simulink model "detumbling1"  (R2022b)
settings: Solver=ode5  StartTime=startTime  StopTime=stopTime  FixedStep=stepsize  RelTol=1e-3
undefined symbols (not defined in the file): a, A_BN0, ARW, c, detumblingkb, detumblingkp, e, EHAccuracy, EHSampleRate, first_detumbling_time_1RW, G, GyroSampleRate, H, h_RW_max, i, inertia1, inertia2, inertia3, Inertia_matrix, Inverse_inertia, Ld, Lw, m, maxdipole, MB, MMnoise, MMSampleRate, mu, n, R_e, rho_d_MB, rho_d_SP, rho_s_MB, rho_s_SP, RRW, SP, theta0, torque_RW_max, w0, wheel_axis
libraries: matrix_library x11, vrlib x10, simulink_extras x4
(part 1 of 3)
settings Model: Creator=Alessandro Cambielli  LastModifiedBy=Alessandro Cambielli

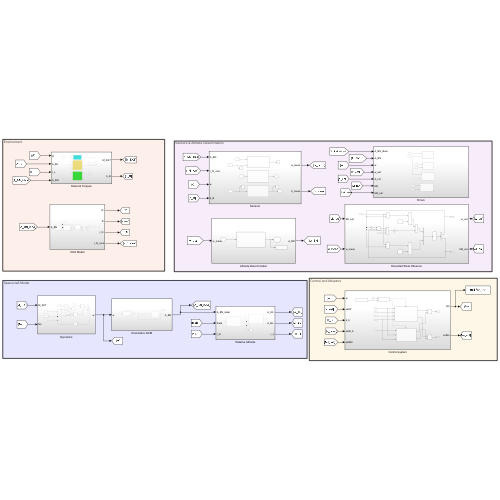
[thumbnail: Simulink's stored preview of the top-level diagram]
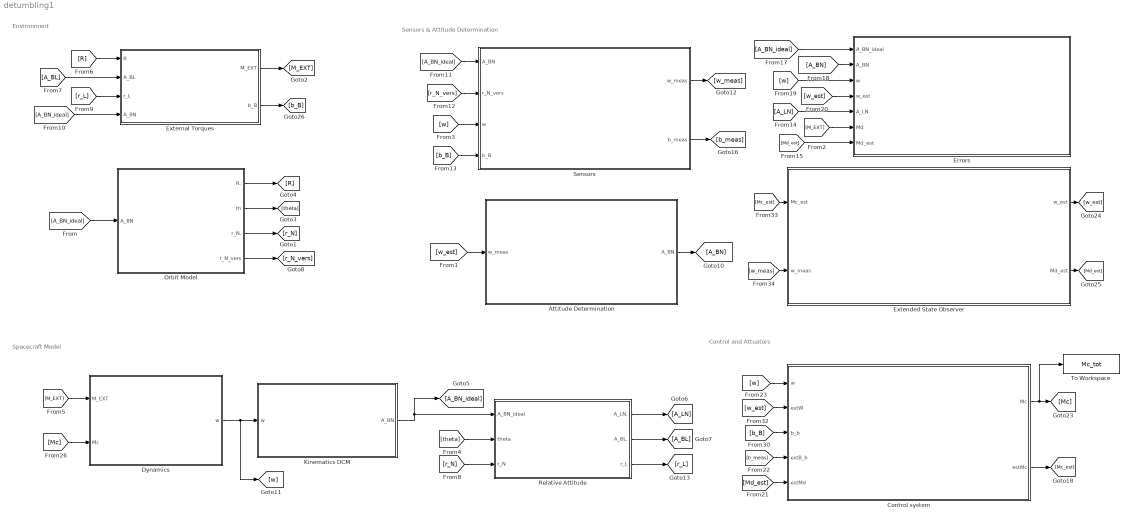
== system detumbling1 ==
  note: Control and Attuators
  note: Sensors & Attitude Determination
  note: Environment
  note: Spacecraft Model
  Attitude Determination : Subsystem
  Control system : Subsystem
  Dynamics : Subsystem
  Errors : Subsystem
  Extended State Observer : Subsystem
  External Torques : Subsystem
  Kinematics DCM : Subsystem
  Orbit Model : Subsystem
  Relative Attitude : Subsystem
  Sensors : Subsystem
  To Workspace : ToWorkspace  VariableName=Mc_tot  SaveFormat=Timeseries  SampleTime=-1
  wires:
  External Torques/2(b_B) -> [b_B]
  [w_est] -> Errors/4(w_est)
  Kinematics DCM/1(A_BN) -> Relative Attitude/1(A_BN_ideal), [A_BN_ideal]
  [w_est] -> Attitude Determination/1(w_meas)
  [M_EXT] -> Errors/6(Md)
  [A_BL] -> External Torques/2(A_BL)
  [Md_est] -> Errors/7(Md_est)
  Orbit Model/3(r_N.) -> [r_N]
  Relative Attitude/2(A_BL.) -> [A_BL]
  Sensors/1(w_meas) -> [w_meas]
  External Torques/1(M_EXT) -> [M_EXT]
  [M_EXT] -> Dynamics/1(M_EXT)
  [A_BN_ideal] -> Orbit Model/1(A_BN)
  Relative Attitude/1(A_LN.) -> [A_LN]
  Sensors/2(b_meas) -> [b_meas]
  [b_B] -> Control system/3(b_b)
  [w_est] -> Control system/2(estW)
  Orbit Model/2(th) -> [theta]
  [A_BN_ideal] -> Errors/1(A_BN_ideal)
  Orbit Model/4(r_N_vers) -> [r_N_vers]
  [r_N_vers] -> Sensors/2(r_N_vers)
  [w_meas] -> Extended State Observer/2(w_meas)
  [r_N] -> Relative Attitude/3(r_N)
  [Md_est] -> Control system/5(estMd)
  Extended State Observer/2(Md_est) -> [Md_est]
  [w] -> Control system/1(w)
  Dynamics/1(w) -> [w], Kinematics DCM/1(w)
  Orbit Model/1(R.) -> [R]
  Control system/2(estMc) -> [Mc_est]
  Control system/1(Mc) -> To Workspace/1, [Mc]
  Relative Attitude/3(r_L) -> [r_L]
  Extended State Observer/1(w_est) -> [w_est]
  [A_BN_ideal] -> Sensors/1(A_BN)
  [A_BN] -> Errors/2(A_BN)
  [A_BN_ideal] -> External Torques/4(A_BN)
  [w] -> Sensors/3(w)
  Attitude Determination/1(A_BN) -> [A_BN]
  [R] -> External Torques/1(R)
  [theta] -> Relative Attitude/2(theta)
  [A_LN] -> Errors/5(A_LN)
  [b_meas] -> Control system/4(estB_b)
  [b_B] -> Sensors/4(b_B)
  [Mc_est] -> Extended State Observer/1(Mc_est)
  [r_L] -> External Torques/3(r_L)
  [w] -> Errors/3(w)
  [Mc] -> Dynamics/2(Mc)

== system detumbling1/Attitude Determination ==
  w_meas : Inport
  Kinematics DCM1 : Subsystem
  To Workspace : ToWorkspace  VariableName=A_BN  SampleTime=-1
  A_BN : Outport
  wires:
  w_meas/1 -> Kinematics DCM1/1(w)
  Kinematics DCM1/1(A_BN) -> To Workspace/1, A_BN/1

== system detumbling1/Control system ==
  w : Inport
  estW : Inport  Port=2
  b_b : Inport  Port=3
  estB_b : Inport  Port=4
  estMd : Inport  Port=5
  Clock : Clock
  Constant : Constant  Value=first_detumbling_time_1RW
  If : If  NumInputs=2  IfExpression=u1 <= u2
  Merge : Merge
  Merge1 : Merge
  Proportional control (RWs) : Subsystem  TreatAsAtomicUnit=on
  Spin rate damping (MT) : Subsystem  TreatAsAtomicUnit=on
  Mc : Outport
  estMc : Outport  Port=2
  wires:
  b_b/1 -> Spin rate damping (MT)/2(b_b)
  Spin rate damping (MT)/1(Mc) -> Merge/1
  Constant/1 -> If/2
  Spin rate damping (MT)/2(estMc) -> Merge1/1
  Proportional control (RWs)/1(Mc) -> Merge/2
  Merge/1 -> Mc/1
  Merge1/1 -> estMc/1
  estB_b/1 -> Spin rate damping (MT)/3(estB_b)
  Clock/1 -> If/1
  estMd/1 -> Proportional control (RWs)/3(estMd), Spin rate damping (MT)/4(estMd)
  If/2 -> Proportional control (RWs)/Action
  estW/1 -> Proportional control (RWs)/2(estW), Spin rate damping (MT)/1(estW)
  If/1 -> Spin rate damping (MT)/Action
  w/1 -> Proportional control (RWs)/1(w)
  Proportional control (RWs)/2(estMc) -> Merge1/2

== system detumbling1/Dynamics ==
  M_EXT : Inport
  Mc : Inport  Port=2
  Constant : Constant  Value=Inverse_inertia
  Constant1 : Constant  Value=Inertia_matrix
  Constant2 : Constant  Value=Inverse_inertia
  Cross Product : matrix_library/Cross Product
  Integrator : Integrator  InitialCondition=w0
  MatrixMultiply : Product  Multiplication=Matrix(*)
  MatrixMultiply1 : Product  Multiplication=Matrix(*)
  MatrixMultiply2 : Product  Multiplication=Matrix(*)
  Scope : Scope
  Sum : Sum
  Sum1 : Sum
  To Workspace : ToWorkspace  VariableName=w  SaveFormat=Timeseries  SampleTime=-1
  w : Outport
  wires:
  MatrixMultiply2/1 -> Sum1/2
  Sum1/1 -> Integrator/1
  Integrator/1 -> w/1, Cross Product/2, Scope/1, To Workspace/1, MatrixMultiply1/2
  Constant/1 -> MatrixMultiply/1
  Constant2/1 -> MatrixMultiply2/1
  MatrixMultiply/1 -> Sum1/1
  Constant1/1 -> MatrixMultiply1/1
  Cross Product/1 -> MatrixMultiply/2
  MatrixMultiply1/1 -> Cross Product/1
  Sum/1 -> MatrixMultiply2/2
  M_EXT/1 -> Sum/1
  Mc/1 -> Sum/2

== system detumbling1/Errors ==
  A_BN_ideal : Inport
  A_BN : Inport  Port=2
  w : Inport  Port=3
  w_est : Inport  Port=4
  A_LN : Inport  Port=5
  Md : Inport  Port=6
  Md_est : Inport  Port=7
  Md error : Subsystem
  Subsystem : Subsystem
  omega error : Subsystem
  pointing error : Subsystem
  wires:
  w/1 -> omega error/1(w)
  w_est/1 -> omega error/2(w_meas)
  A_BN_ideal/1 -> Subsystem/1(A_BN_ideal)
  A_BN/1 -> Subsystem/2(A_BN), pointing error/1(A_BN)
  A_LN/1 -> pointing error/2(A_LN)
  Md/1 -> Md error/1(Md)
  Md_est/1 -> Md error/2(Md_est)

== system detumbling1/Extended State Observer ==
  Mc_est : Inport
  w_meas : Inport  Port=2
  Constant4 : Constant  Value=Lw
  Constant5 : Constant  Value=Ld
  Cross Product : vrlib/Utilities/Cross Product
  Demux1 : Demux  Outputs=2
  Gain : Gain  Gain=Inertia_matrix  Multiplication=Matrix(K*u)
  Gain1 : Gain  Gain=Inverse_inertia  Multiplication=Matrix(K*u)
  Integrator : Integrator  InitialCondition=[w0; [0; 0; 0]]
  Mux : Mux  Inputs=2
  Product4 : Product
  Product5 : Product
  Sum4 : Sum  Inputs=+-
  Sum5 : Sum  Inputs=+-
  Sum6 : Sum
  Sum7 : Sum  Inputs=+++
  w_est : Outport
  Md_est : Outport  Port=2
  wires:
  Gain/1 -> Cross Product/1
  Sum5/1 -> Product5/1
  Constant5/1 -> Product5/2
  Cross Product/1 -> Sum7/1
  Product5/1 -> Mux/2
  Demux1/1 -> Sum5/2, Cross Product/2, Gain/1, Sum4/2, w_est/1
  Sum7/1 -> Gain1/1
  Gain1/1 -> Sum6/2
  Product4/1 -> Sum6/1
  Sum6/1 -> Mux/1
  Demux1/2 -> Md_est/1, Sum7/2
  Mux/1 -> Integrator/1
  Mc_est/1 -> Sum7/3
  w_meas/1 -> Sum5/1, Sum4/1
  Integrator/1 -> Demux1/1
  Constant4/1 -> Product4/2
  Sum4/1 -> Product4/1

== system detumbling1/External Torques ==
  R : Inport
  A_BL : Inport  Port=2
  r_L : Inport  Port=3
  A_BN : Inport  Port=4
  Constant : Constant  Value=MB
  Constant1 : Constant  Value=SP
  M_GG : Subsystem
  Magnetic field : Subsystem
  Solar radiation : Subsystem
  Sum of Elements : Sum  Inputs=+++
  To Workspace : ToWorkspace  VariableName=M_GG  SaveFormat=Timeseries  SampleTime=-1
  To Workspace1 : ToWorkspace  VariableName=M_SRP  SaveFormat=Timeseries  SampleTime=-1
  To Workspace2 : ToWorkspace  VariableName=M_MAG  SaveFormat=Timeseries  SampleTime=-1
  M_EXT : Outport
  b_B : Outport  Port=2
  wires:
  [R] -> M_GG/2(R)
  Constant/1 -> Solar radiation/2(MB)
  Constant1/1 -> Solar radiation/3(SP)
  [A_BN] -> Solar radiation/1(A_BN)
  [A_BN] -> Magnetic field/2(A_BN)
  Magnetic field/1(M_MAG) -> Sum of Elements/3, To Workspace2/1
  Sum of Elements/1 -> M_EXT/1
  [A_BL] -> M_GG/1(A_BL)
  [r_L] -> Magnetic field/1(r_L)
  R/1 -> [R]
  A_BL/1 -> [A_BL]
  M_GG/1(M_GG1) -> Sum of Elements/1, To Workspace/1
  r_L/1 -> [r_L]
  A_BN/1 -> [A_BN]
  Solar radiation/1(T_SRP) -> To Workspace1/1, Sum of Elements/2
  Magnetic field/2(b_B) -> b_B/1

== system detumbling1/Kinematics DCM ==
  w : Inport
  Gain : Gain  Gain=-1
  Integrator : Integrator  InitialCondition=A_BN0
  Product : Product  Multiplication=Matrix(*)
  To Workspace : ToWorkspace  VariableName=A_BN_ideal  SampleTime=-1
  orthonormalization : Subsystem
  w_cross : Subsystem
  A_BN : Outport
  wires:
  w_cross/1(w_cross) -> Gain/1
  Product/1 -> Integrator/1
  Gain/1 -> Product/1
  Integrator/1 -> orthonormalization/1(A0(t))
  orthonormalization/1(A(t)) -> A_BN/1, To Workspace/1, Product/2
  w/1 -> w_cross/1(w)

== system detumbling1/Orbit Model ==
  A_BN : Inport
  Normalize Vector : vrlib/Utilities/Normalize Vector  maxzero=0
  Product : Product  Multiplication=Matrix(*)
  R : Subsystem
  To Workspace1 : ToWorkspace  VariableName=r_B_vers  SampleTime=-1
  r_N : Subsystem
  theta : Subsystem
  R. : Outport
  th : Outport  Port=2
  r_N. : Outport  Port=3
  r_N_vers : Outport  Port=4
  wires:
  Normalize Vector/1 -> r_N_vers/1, Product/2
  r_N/1(r_N) -> r_N./1, Normalize Vector/1
  R/1(R) -> R./1, r_N/2(R)
  Product/1 -> To Workspace1/1
  theta/1(theta) -> th/1, r_N/1(theta), R/1(theta)
  A_BN/1 -> Product/1

== system detumbling1/Relative Attitude ==
  A_BN_ideal : Inport
  theta : Inport  Port=2
  r_N : Inport  Port=3
  A_BL : Subsystem
  A_LN : Subsystem
  MatrixMultiply : Product  Multiplication=Matrix(*)
  A_LN. : Outport
  A_BL. : Outport  Port=2
  r_L : Outport  Port=3
  wires:
  A_LN/1(A_LN) -> MatrixMultiply/1, A_LN./1, A_BL/2(A_LN)
  theta/1 -> A_LN/1(theta)
  A_BN_ideal/1 -> A_BL/1(A_BN)
  A_BL/1(A_BL) -> A_BL./1
  r_N/1 -> MatrixMultiply/2
  MatrixMultiply/1 -> r_L/1

== system detumbling1/Sensors ==
  A_BN : Inport
  r_N_vers : Inport  Port=2
  w : Inport  Port=3
  b_B : Inport  Port=4
  Earth Horizon Sensor : Subsystem
  Gyroscope : Subsystem
  Magnetometer : Subsystem
  Scope{,1..3} (4 alike) : Scope
  w_meas : Outport
  b_meas : Outport  Port=2
  wires:
  A_BN/1 -> Earth Horizon Sensor/1(A_BN)
  r_N_vers/1 -> Scope/1, Earth Horizon Sensor/2(r_N_vers)
  w/1 -> Gyroscope/1(w)
  b_B/1 -> Scope2/1, Magnetometer/1(b_B)
  Earth Horizon Sensor/1(EH_meas) -> Scope1/1
  Gyroscope/1(w_meas) -> w_meas/1
  Magnetometer/1(MM_meas) -> Scope3/1, b_meas/1

== system detumbling1/Attitude Determination/Kinematics DCM1 ==
  w : Inport
  Gain : Gain  Gain=-1
  Integrator : Integrator  InitialCondition=A_BN0
  Product : Product  Multiplication=Matrix(*)
  orthonormalization : Subsystem
  w_cross : Subsystem
  A_BN : Outport
  wires:
  w_cross/1(w_cross) -> Gain/1
  Product/1 -> Integrator/1
  Gain/1 -> Product/1
  Integrator/1 -> orthonormalization/1(A0(t))
  orthonormalization/1(A(t)) -> A_BN/1, Product/2
  w/1 -> w_cross/1(w)

== system detumbling1/Control system/Proportional control (RWs) ==
  w : Inport
  estW : Inport  Port=2
  estMd : Inport  Port=3
  Action Port : ActionPort  ActionPortLabel=else
  Ideal control law : Subsystem  TreatAsAtomicUnit=on
  Reaction wheels : Subsystem
  Scope : Scope
  To Workspace : ToWorkspace  VariableName=Mc_RW  SaveFormat=Timeseries  SampleTime=-1
  Mc : Outport
  estMc : Outport  Port=2
  wires:
  Reaction wheels/2(estMc_RW) -> estMc/1
  Ideal control law/1(Mc_id) -> Reaction wheels/1(targetMc)
  w/1 -> Reaction wheels/2(w)
  estW/1 -> Reaction wheels/3(estW), Ideal control law/1(estW)
  estMd/1 -> Ideal control law/2(estMd)
  Reaction wheels/1(Mc_RW) -> To Workspace/1, Scope/1, Mc/1

== system detumbling1/Control system/Spin rate damping (MT) ==
  estW : Inport
  b_b : Inport  Port=2
  estB_b : Inport  Port=3
  estMd : Inport  Port=4
  Action Port : ActionPort  ActionPortLabel=if(u1 <= u2)
  Ideal control law : Subsystem
  Magnetorquer : Subsystem
  Scope : Scope
  To Workspace : ToWorkspace  VariableName=Mc_MT  SaveFormat=Timeseries  SampleTime=-1
  Mc : Outport
  estMc : Outport  Port=2
  wires:
  b_b/1 -> Magnetorquer/2(b_b)
  estB_b/1 -> Magnetorquer/3(estB_b), Ideal control law/2(estB_b)
  Ideal control law/1(targetMc) -> Magnetorquer/1(targetMc)
  Magnetorquer/1(Mc_MT) -> Scope/1, To Workspace/1, Mc/1
  estMd/1 -> Ideal control law/3(estMd)
  estW/1 -> Ideal control law/1(estW)
  Magnetorquer/2(estMc_MT) -> estMc/1

== system detumbling1/Errors/Md error ==
  Md : Inport
  Md_est : Inport  Port=2
  Scope2 : Scope
  Sum : Sum  Inputs=+-
  To Workspace1 : ToWorkspace  VariableName=delta_Md  SaveFormat=Timeseries  SampleTime=-1
  wires:
  Sum/1 -> Scope2/1, To Workspace1/1
  Md/1 -> Sum/1
  Md_est/1 -> Sum/2

== system detumbling1/Errors/Subsystem ==
  A_BN_ideal : Inport
  A_BN : Inport  Port=2
  Acos : Trigonometry  Commented=on  Operator=acos
  Acos1 : Trigonometry  Commented=on  Operator=acos
  Constant : Constant  Value=eye(3)
  Gain : Gain  Commented=on  Gain=2
  Gain1 : Gain  Commented=on  Gain=2
  MATLAB Function : MATLAB Function  Commented=on  TreatAsAtomicUnit=on
  MatrixMultiply : Product  Multiplication=Matrix(*)
  Radians to Degrees : simulink_extras/Transformations/Radians to Degrees  Commented=on
  Radians to Degrees1 : simulink_extras/Transformations/Radians to Degrees  Commented=on
  Sum : Sum  Inputs=+-
  Sum1 : Sum  Commented=on  Inputs=+-
  To Workspace : ToWorkspace  VariableName=A_error  SaveFormat=Timeseries  SampleTime=-1
  Transpose : Math  Operator=transpose
  wires:
  MATLAB Function/1(q4) -> Acos/1
  MATLAB Function/2(q4_sens) -> Acos1/1
  Acos/1 -> Gain/1
  Acos1/1 -> Gain1/1
  Gain/1 -> Radians to Degrees/1
  Gain1/1 -> Radians to Degrees1/1
  Radians to Degrees/1 -> Sum1/1
  Radians to Degrees1/1 -> Sum1/2
  A_BN_ideal/1 -> MatrixMultiply/1
  A_BN/1 -> Transpose/1
  Transpose/1 -> MatrixMultiply/2
  MatrixMultiply/1 -> Sum/1
  Constant/1 -> Sum/2
  Sum/1 -> To Workspace/1

== system detumbling1/Errors/omega error ==
  w : Inport
  w_meas : Inport  Port=2
  Scope : Scope
  Sum1 : Sum  Inputs=+-
  To Workspace1 : ToWorkspace  VariableName=delta_omega  SaveFormat=Timeseries  SampleTime=-1
  wires:
  Sum1/1 -> Scope/1, To Workspace1/1
  w/1 -> Sum1/1
  w_meas/1 -> Sum1/2

== system detumbling1/Errors/pointing error ==
  A_BN : Inport
  A_LN : Inport  Port=2
  Constant : Constant  Value=[1; 0; 0]
  Constant1 : Constant  Value=[1; 0; 0]
  Dot Product : DotProduct  OutDataTypeStr=Inherit: Inherit via internal rule
  MatrixMultiply : Product  Inputs=3  Multiplication=Matrix(*)
  Radians to Degrees : simulink_extras/Transformations/Radians to Degrees
  Scope : Scope
  To Workspace : ToWorkspace  VariableName=point_error  SaveFormat=Timeseries  SampleTime=-1
  Transpose1 : matrix_library/Transpose
  Trigonometric Function : Trigonometry  Operator=acos
  wires:
  A_LN/1 -> Transpose1/1
  Trigonometric Function/1 -> Radians to Degrees/1
  A_BN/1 -> MatrixMultiply/1
  Transpose1/1 -> MatrixMultiply/2
  Constant/1 -> MatrixMultiply/3
  MatrixMultiply/1 -> Dot Product/1
  Constant1/1 -> Dot Product/2
  Dot Product/1 -> Trigonometric Function/1
  Radians to Degrees/1 -> Scope/1, To Workspace/1

== system detumbling1/External Torques/M_GG ==
  A_BL : Inport
  R : Inport  Port=2
  GG Torque1 : Subsystem
  "c1, c2, c3" : Subsystem
  M_GG1 : Outport
  wires:
  "c1, c2, c3"/1(c1) -> GG Torque1/1(c1)
  "c1, c2, c3"/2(c2) -> GG Torque1/2(c2)
  "c1, c2, c3"/3(c3) -> GG Torque1/3(c3)
  A_BL/1 -> "c1, c2, c3"/1(A_BL)
  GG Torque1/1(M_GG) -> M_GG1/1
  R/1 -> GG Torque1/4(R)

== system detumbling1/External Torques/Magnetic field ==
  r_L : Inport
  A_BN : Inport  Port=2
  Clock : Clock
  Constant : Constant  Value=m
  Constant1 : Constant  Value=R_e*1000
  Constant3 : Constant  Value=G
  Constant4 : Constant  Value=H
  Cross Product1 : matrix_library/Cross Product
  MATLAB Function : MATLAB Function  TreatAsAtomicUnit=on
  MatrixMultiply : Product  Multiplication=Matrix(*)
  Reshape1 : Reshape  OutputDimensionality=Column vector (2-D)
  M_MAG : Outport
  b_B : Outport  Port=2
  wires:
  Constant1/1 -> MATLAB Function/2(r)
  Clock/1 -> MATLAB Function/3(t)
  Constant3/1 -> MATLAB Function/4(G)
  MATLAB Function/1(b_N) -> Reshape1/1
  r_L/1 -> MATLAB Function/1(r_LVLH)
  Reshape1/1 -> MatrixMultiply/2
  Constant4/1 -> MATLAB Function/5(H)
  A_BN/1 -> MatrixMultiply/1
  Constant/1 -> Cross Product1/1
  MatrixMultiply/1 -> b_B/1, Cross Product1/2
  Cross Product1/1 -> M_MAG/1

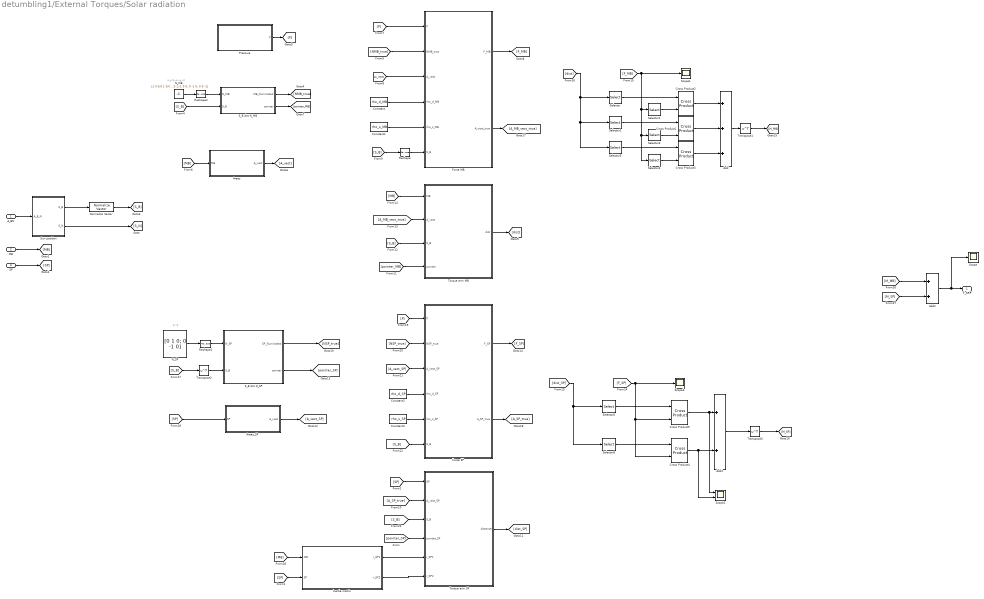
== system detumbling1/External Torques/Solar radiation ==
  note: x,y,z,-x,-y,-z
  note: y,-y
  A_BN : Inport
  MB : Inport  Port=2
  SP : Inport  Port=3
  Add : Sum  Inputs=3
  Add1 : Sum
  Add2 : Sum
  Areas : Subsystem
  Areas_SP : Subsystem
  Constant : Constant  Value=rho_d_MB
  Constant1 : Constant  Value=rho_s_MB
  Constant2 : Constant  Value=rho_d_SP
  Constant3 : Constant  Value=rho_s_SP
  Cross Product{1..5} (5 alike) : matrix_library/Cross Product
  Force MB : Subsystem
  Force SP : Subsystem
  Inertia matrix : Subsystem
  N_MB : Constant  Value=[1 0 0;0 1 0;0 0 1;-1 0 0; 0 -1 0; 0 0 -1]  VectorParams1D=off
  N_SP : Constant  Value=[0 1 0; 0 -1 0]  VectorParams1D=off
  Normalize Vector : vrlib/Utilities/Normalize Vector  maxzero=0
  Pressure : Subsystem
  Reshape : Reshape  OutputDimensionality=Column vector (2-D)
  Reshape1 : Reshape  OutputDimensionality=Customize  OutputDimensions=[2,3]
  Reshape2 : Reshape  OutputDimensionality=Customize  OutputDimensions=[6,3]
  S_B dot N_MB : Subsystem
  S_B dot N_SP : Subsystem
  Scope : Scope
  Scope1 : Scope
  Scope2 : Scope  NumInputPorts=2
  Scope3 : Scope
  Selector : Selector  NumberOfDimensions=2  InputPortWidth=3  IndexOptions=Index vector (dialog),Index vector (dialog)  Indices=1,[1 2 3]  OutputSizes=1,1
  Selector1 : Selector  NumberOfDimensions=2  InputPortWidth=3  IndexOptions=Index vector (dialog),Index vector (dialog)  Indices=1,[1 2 3]  OutputSizes=1,1
  Selector2 : Selector  NumberOfDimensions=2  InputPortWidth=3  IndexOptions=Index vector (dialog),Index vector (dialog)  Indices=2,[1 2 3]  OutputSizes=1,1
  Selector3 : Selector  NumberOfDimensions=2  InputPortWidth=3  IndexOptions=Index vector (dialog),Index vector (dialog)  Indices=2,[1 2 3]  OutputSizes=1,1
  Selector4 : Selector  NumberOfDimensions=2  InputPortWidth=3  IndexOptions=Index vector (dialog),Index vector (dialog)  Indices=3,[1 2 3]  OutputSizes=1,1
  Selector5 : Selector  NumberOfDimensions=2  InputPortWidth=3  IndexOptions=Index vector (dialog),Index vector (dialog)  Indices=3,[1 2 3]  OutputSizes=1,1
  Selector6 : Selector  NumberOfDimensions=2  InputPortWidth=3  IndexOptions=Index vector (dialog),Index vector (dialog)  Indices=1,[1 2 3]  OutputSizes=1,1
  Selector8 : Selector  NumberOfDimensions=2  InputPortWidth=3  IndexOptions=Index vector (dialog),Index vector (dialog)  Indices=2,[1 2 3]  OutputSizes=1,1
  Sun position : Subsystem
  Torque arm MB : Subsystem
  Torque arm SP : Subsystem
  Transpose1 : Math  Operator=transpose
  Transpose2 : Math  Operator=transpose
  Transpose3 : Math  Operator=transpose
  T_SRP : Outport
  wires:
  Sun position/1(S_B) -> Normalize Vector/1
  MB/1 -> [MB]
  N_MB/1 -> Reshape2/1
  [NMB_true] -> Force MB/2(NMB_true)
  S_B dot N_MB/1(MB_illuminated) -> [NMB_true]
  [MB] -> Areas/1(MB)
  [S_B] -> S_B dot N_MB/2(S_B)
  Sun position/2(S_N) -> [S_N]
  [P] -> Force MB/1(P)
  Areas/1(A_vect) -> [A_vect]
  Transpose1/1 -> [M_MB]
  Areas_SP/1(A_vect) -> [A_vect_SP]
  Reshape1/1 -> S_B dot N_SP/1(N_SP)
  Transpose3/1 -> [M_SP]
  Selector2/1 -> Cross Product1/1
  [MB] -> Torque arm MB/1(MB)
  Constant3/1 -> Force SP/5(rho_s_SP)
  [F_SP] -> Cross Product5/2, Cross Product4/2, Scope3/1
  [M_MB] -> Add2/1
  [dist_SP] -> Selector6/1, Selector8/1
  [pointer_SP] -> Torque arm SP/4(pointer_SP)
  Cross Product4/1 -> Scope2/2, Add1/2
  [F_MB] -> Scope1/1, Selector4/1, Selector3/1, Selector1/1
  A_BN/1 -> Sun position/1(A_B_N)
  Add1/1 -> Transpose3/1
  Transpose2/1 -> S_B dot N_SP/2(S_B)
  [SP] -> Areas_SP/1(SP)
  [A_SP_true] -> Torque arm SP/2(A_vect_SP)
  Add/1 -> Transpose1/1
  Torque arm SP/1(distance) -> [dist_SP]
  Reshape2/1 -> S_B dot N_MB/1(N_MB)
  Torque arm MB/1(dist) -> [dist]
  S_B dot N_SP/2(pointer) -> [pointer_SP]
  Force MB/1(F_MB) -> [F_MB]
  Selector/1 -> Cross Product2/1
  [S_B] -> Reshape/1
  [P] -> Force SP/1(P)
  [A_vect] -> Force MB/3(A_vect)
  Selector1/1 -> Cross Product2/2
  Constant1/1 -> Force MB/5(rho_s_MB)
  [A_MB_vect_true] -> Torque arm MB/2(A_vect)
  Pressure/1(P) -> [P]
  Normalize Vector/1 -> [S_B]
  Constant2/1 -> Force SP/4(rho_d_SP)
  Constant/1 -> Force MB/4(rho_d_MB)
  Selector8/1 -> Cross Product4/1
  [dist] -> Selector2/1, Selector5/1, Selector/1
  [NSP_true] -> Force SP/2(NSP_true)
  N_SP/1 -> Reshape1/1
  [S_B] -> Torque arm MB/3(S_B)
  Force SP/2(A_SP_true) -> [A_SP_true]
  [S_B] -> Torque arm SP/3(S_B)
  SP/1 -> [SP]
  Selector4/1 -> Cross Product3/2
  S_B dot N_MB/2(pointer) -> [pointer_MB]
  Force MB/2(A_vect_true) -> [A_MB_vect_true]
  [pointer_MB] -> Torque arm MB/4(pointer)
  Add2/1 -> Scope/1, T_SRP/1
  Selector3/1 -> Cross Product1/2
  [S_B] -> Force SP/6(S_B)
  [S_B] -> Transpose2/1
  Cross Product5/1 -> Scope2/1, Add1/1
  [A_vect_SP] -> Force SP/3(A_vect_SP)
  Reshape/1 -> Force MB/6(S_B)
  Cross Product2/1 -> Add/1
  Force SP/1(F_SP) -> [F_SP]
  S_B dot N_SP/1(SP_illuminated) -> [NSP_true]
  Selector6/1 -> Cross Product5/1
  Selector5/1 -> Cross Product3/1
  Cross Product1/1 -> Add/2
  [M_SP] -> Add2/2
  [SP] -> Torque arm SP/1(SP)
  Cross Product3/1 -> Add/3
  [SP] -> Inertia matrix/2(SP)
  [MB] -> Inertia matrix/1(MB)
  Inertia matrix/1(r_SP1) -> Torque arm SP/5(r_SP1)
  Inertia matrix/2(r_SP2) -> Torque arm SP/6(r_SP2)

== system detumbling1/Kinematics DCM/orthonormalization ==
  A0(t) : Inport
  Gain : Gain  Gain=3/2
  Gain1 : Gain  Gain=0.5
  Product : Product  Inputs=3  Multiplication=Matrix(*)
  Sum : Sum  Inputs=+-
  Transpose : matrix_library/Transpose
  A(t) : Outport
  wires:
  Sum/1 -> A(t)/1
  Product/1 -> Sum/2
  Gain1/1 -> Product/3
  Transpose/1 -> Product/2
  A0(t)/1 -> Product/1, Gain/1, Gain1/1, Transpose/1
  Gain/1 -> Sum/1

== system detumbling1/Kinematics DCM/w_cross ==
  w : Inport
  Constant : Constant  Value=0
  Display : Display
  Gain : Gain  Gain=[1; 1; -1]
  Gain1 : Gain  Gain=[-1; 1; 1]
  Gain2 : Gain  Gain=[1; -1; 1]
  Matrix Concatenate : Concatenate  NumInputs=3  Mode=Multidimensional array  ConcatenateDimension=2
  Selector : Selector  InputPortWidth=4  IndexOptions=Index vector (dialog)  Indices=[1, 4, 3]  OutputSizes=1
  Selector1 : Selector  InputPortWidth=4  IndexOptions=Index vector (dialog)  Indices=[4, 1, 2]  OutputSizes=1
  Selector2 : Selector  InputPortWidth=4  IndexOptions=Index vector (dialog)  Indices=[3, 2, 1]  OutputSizes=1
  Vector Concatenate : Concatenate
  w_cross : Outport
  wires:
  Matrix Concatenate/1 -> w_cross/1, Display/1
  Vector Concatenate/1 -> Selector2/1, Selector/1, Selector1/1
  Selector2/1 -> Gain2/1
  Selector/1 -> Gain/1
  Constant/1 -> Vector Concatenate/1
  Selector1/1 -> Gain1/1
  Gain2/1 -> Matrix Concatenate/3
  Gain1/1 -> Matrix Concatenate/2
  Gain/1 -> Matrix Concatenate/1
  w/1 -> Vector Concatenate/2

== system detumbling1/Orbit Model/R ==
  theta : Inport
  Constant : Constant  Value=a
  Constant1 : Constant  Value=1-e^2
  Constant2 : Constant
  Constant3 : Constant  Value=e
  Cos : Trigonometry  Operator=cos
  Divide : Product  Inputs=*/
  Product : Product
  Product1 : Product
  Sum : Sum
  R : Outport
  wires:
  Sum/1 -> Divide/2
  Constant/1 -> Product/1
  Constant2/1 -> Sum/1
  Cos/1 -> Product1/2
  Product/1 -> Divide/1
  theta/1 -> Cos/1
  Divide/1 -> R/1
  Product1/1 -> Sum/2
  Constant3/1 -> Product1/1
  Constant1/1 -> Product/2

== system detumbling1/Orbit Model/r_N ==
  theta : Inport
  R : Inport  Port=2
  Constant : Constant  Value=cos(i)
  Constant1 : Constant  Value=sin(i)
  Cos : Trigonometry  Operator=cos
  Mux : Mux  Inputs=3
  Product : Product
  Product1 : Product
  Product2 : Product
  Sin : Trigonometry
  Sin1 : Trigonometry
  r_N : Outport
  wires:
  Constant/1 -> Product/2
  Cos/1 -> Mux/1
  Product/1 -> Mux/2
  Sin/1 -> Product/1
  Constant1/1 -> Product1/2
  Sin1/1 -> Product1/1
  Product1/1 -> Mux/3
  theta/1 -> Sin1/1, Cos/1, Sin/1
  Mux/1 -> Product2/2
  R/1 -> Product2/1
  Product2/1 -> r_N/1

== system detumbling1/Orbit Model/theta ==
  Constant : Constant
  Constant1 : Constant  Value=e
  Constant2 : Constant  Value=2
  Constant3 : Constant  Value=1-e^2
  Constant4 : Constant  Value=3/2
  Constant5 : Constant  Value=n
  Cos : Trigonometry  Operator=cos
  Divide : Product  Inputs=*/
  Integrator : Integrator  InitialCondition=theta0
  Pow : Math  Operator=pow  RndMeth=Zero
  Pow1 : Math  Operator=pow  RndMeth=Zero
  Product : Product
  Product1 : Product
  Sum : Sum
  To Workspace : ToWorkspace  VariableName=theta  SampleTime=-1
  theta : Outport
  wires:
  Cos/1 -> Product/2
  Constant/1 -> Sum/1
  Product/1 -> Sum/2
  Constant2/1 -> Pow/2
  Sum/1 -> Pow/1
  Constant1/1 -> Product/1
  Pow/1 -> Product1/2
  Product1/1 -> Divide/1
  Constant3/1 -> Pow1/1
  Constant4/1 -> Pow1/2
  Pow1/1 -> Divide/2
  Divide/1 -> Integrator/1
  Integrator/1 -> To Workspace/1, theta/1, Cos/1
  Constant5/1 -> Product1/1

== system detumbling1/Relative Attitude/A_BL ==
  A_BN : Inport
  A_LN : Inport  Port=2
  Matrix Multiply : Product  Multiplication=Matrix(*)
  To Workspace : ToWorkspace  VariableName=A_BL  SampleTime=-1
  Transpose1 : matrix_library/Transpose
  A_BL : Outport
  wires:
  A_BN/1 -> Matrix Multiply/1
  A_LN/1 -> Transpose1/1
  Transpose1/1 -> Matrix Multiply/2
  Matrix Multiply/1 -> A_BL/1, To Workspace/1

== system detumbling1/Relative Attitude/A_LN ==
  theta : Inport
  Constant : Constant  Value=0
  Constant1 : Constant  Value=[0; 0; 1]
  Constant2 : Constant  Value=[1 0 0; 0 cos(i) sin(i); 0 -sin(i) cos(i)]
  Cos : Trigonometry  Operator=cos
  Gain : Gain  Gain=[1; -1; 1]
  Matrix Concatenate : Concatenate  NumInputs=3  Mode=Multidimensional array  ConcatenateDimension=2
  Product : Product  Multiplication=Matrix(*)
  Selector : Selector  InputPortWidth=3  IndexOptions=Index vector (dialog)  Indices=[3 2 1]  OutputSizes=1
  Selector1 : Selector  InputPortWidth=3  IndexOptions=Index vector (dialog)  Indices=[2 3 1]  OutputSizes=1
  Sin : Trigonometry
  To Workspace : ToWorkspace  VariableName=A_LN  SampleTime=-1
  Vector Concatenate : Concatenate  NumInputs=3
  A_LN : Outport
  wires:
  Matrix Concatenate/1 -> Product/1
  theta/1 -> Sin/1, Cos/1
  Gain/1 -> Matrix Concatenate/1
  Vector Concatenate/1 -> Selector1/1, Selector/1
  Sin/1 -> Vector Concatenate/3
  Selector/1 -> Matrix Concatenate/2
  Selector1/1 -> Gain/1
  Product/1 -> A_LN/1, To Workspace/1
  Constant1/1 -> Matrix Concatenate/3
  Cos/1 -> Vector Concatenate/2
  Constant/1 -> Vector Concatenate/1
  Constant2/1 -> Product/2

== system detumbling1/Sensors/Earth Horizon Sensor ==
  A_BN : Inport
  r_N_vers : Inport  Port=2
  A_eps : Subsystem
  MatrixMultiply : Product  Inputs=3  Multiplication=Matrix(*)
  EH_meas : Outport
  wires:
  A_eps/1(A_epsHS) -> MatrixMultiply/1
  A_BN/1 -> MatrixMultiply/2
  r_N_vers/1 -> MatrixMultiply/3
  MatrixMultiply/1 -> EH_meas/1

== system detumbling1/Sensors/Gyroscope ==
  w : Inport
  Integrator : Integrator
  Sum : Sum  Inputs=+++
  db : RandomNumber  Variance=(deg2rad(RRW)/3600/sqrt(1/GyroSampleRate))^2* [1;1;1]  SampleTime=1/GyroSampleRate
  n : RandomNumber  Variance=(deg2rad(ARW)/sqrt(3600)/sqrt(1/GyroSampleRate))^2*[1;1;1]  SampleTime=1/GyroSampleRate
  w_meas : Outport
  wires:
  db/1 -> Integrator/1
  n/1 -> Sum/2
  Integrator/1 -> Sum/3
  w/1 -> Sum/1
  Sum/1 -> w_meas/1

== system detumbling1/Sensors/Magnetometer ==
  b_B : Inport
  Constant : Constant  Value=MMnoise
  MatrixMultiply : Product  Multiplication=Matrix(*)
  Subsystem : Subsystem
  Sum : Sum
  MM_meas : Outport
  wires:
  Constant/1 -> Sum/2
  b_B/1 -> Sum/1  "b_B"
  Subsystem/1(A_epsMM) -> MatrixMultiply/1
  Sum/1 -> MatrixMultiply/2
  MatrixMultiply/1 -> MM_meas/1

== system detumbling1/Attitude Determination/Kinematics DCM1/orthonormalization ==
  A0(t) : Inport
  Gain : Gain  Gain=3/2
  Gain1 : Gain  Gain=0.5
  Product : Product  Inputs=3  Multiplication=Matrix(*)
  Sum : Sum  Inputs=+-
  Transpose : matrix_library/Transpose
  A(t) : Outport
  wires:
  Sum/1 -> A(t)/1
  Product/1 -> Sum/2
  Gain1/1 -> Product/3
  Transpose/1 -> Product/2
  A0(t)/1 -> Product/1, Gain/1, Gain1/1, Transpose/1
  Gain/1 -> Sum/1

== system detumbling1/Attitude Determination/Kinematics DCM1/w_cross ==
  w : Inport
  Constant : Constant  Value=0
  Display : Display
  Gain : Gain  Gain=[1; 1; -1]
  Gain1 : Gain  Gain=[-1; 1; 1]
  Gain2 : Gain  Gain=[1; -1; 1]
  Matrix Concatenate : Concatenate  NumInputs=3  Mode=Multidimensional array  ConcatenateDimension=2
  Selector : Selector  InputPortWidth=4  IndexOptions=Index vector (dialog)  Indices=[1, 4, 3]  OutputSizes=1
  Selector1 : Selector  InputPortWidth=4  IndexOptions=Index vector (dialog)  Indices=[4, 1, 2]  OutputSizes=1
  Selector2 : Selector  InputPortWidth=4  IndexOptions=Index vector (dialog)  Indices=[3, 2, 1]  OutputSizes=1
  Vector Concatenate : Concatenate
  w_cross : Outport
  wires:
  Matrix Concatenate/1 -> w_cross/1, Display/1
  Vector Concatenate/1 -> Selector2/1, Selector/1, Selector1/1
  Selector2/1 -> Gain2/1
  Selector/1 -> Gain/1
  Constant/1 -> Vector Concatenate/1
  Selector1/1 -> Gain1/1
  Gain2/1 -> Matrix Concatenate/3
  Gain1/1 -> Matrix Concatenate/2
  Gain/1 -> Matrix Concatenate/1
  w/1 -> Vector Concatenate/2

== system detumbling1/Control system/Proportional control (RWs)/Ideal control law ==
  estW : Inport
  estMd : Inport  Port=2
  Add : Sum  Inputs=+-
  Gain : Gain  Gain=-detumblingkp
  Mc_id : Outport
  wires:
  estW/1 -> Gain/1
  Gain/1 -> Add/1
  Add/1 -> Mc_id/1
  estMd/1 -> Add/2

== system detumbling1/Control system/Proportional control (RWs)/Reaction wheels ==
  targetMc : Inport
  w : Inport  Port=2
  estW : Inport  Port=3
  Add{,1..3} (4 alike) : Sum  Inputs=--
  Constant{,1..5} (6 alike) : Constant  Value=wheel_axis
  Cross Product : vrlib/Utilities/Cross Product
  Cross Product1 : vrlib/Utilities/Cross Product
  Dot Product : DotProduct  OutDataTypeStr=Inherit: Inherit via internal rule
  Dot Product1 : DotProduct  OutDataTypeStr=Inherit: Inherit via internal rule
  Integrator : Integrator
  Integrator1 : Integrator
  Product{,1..3} (4 alike) : Product
  Saturation : Saturate  UpperLimit=h_RW_max  LowerLimit=-h_RW_max
  Saturation1 : Saturate  UpperLimit=h_RW_max  LowerLimit=-h_RW_max
  Saturation2 : Saturate  UpperLimit=torque_RW_max  LowerLimit=-torque_RW_max
  Saturation3 : Saturate  UpperLimit=torque_RW_max  LowerLimit=-torque_RW_max
  To Workspace : ToWorkspace  VariableName=hr  SampleTime=-1
  Mc_RW : Outport
  estMc_RW : Outport  Port=2
  wires:
  Cross Product/1 -> Add1/1, Add/2
  Add2/1 -> Dot Product1/1
  Integrator/1 -> Saturation/1  "hr"
  Add1/1 -> Saturation2/1
  Product2/1 -> Add3/2
  Add/1 -> Dot Product/1
  Integrator1/1 -> Saturation1/1  "hr"
  targetMc/1 -> Add/1, Add2/1
  Add3/1 -> Saturation3/1
  Cross Product1/1 -> Add3/1, Add2/2
  estW/1 -> Cross Product1/1
  w/1 -> Cross Product/1
  Saturation/1 -> Product1/1, To Workspace/1
  Saturation1/1 -> Product3/1
  Saturation3/1 -> estMc_RW/1
  Saturation2/1 -> Mc_RW/1
  Dot Product/1 -> Product/2, Integrator/1  "hr_dot"
  Constant/1 -> Dot Product/2
  Product/1 -> Add1/2
  Constant1/1 -> Product/1
  Product1/1 -> Cross Product/2
  Constant2/1 -> Product1/2
  Constant3/1 -> Dot Product1/2
  Dot Product1/1 -> Product2/2, Integrator1/1  "hr_dot"
  Constant4/1 -> Product2/1
  Constant5/1 -> Product3/2
  Product3/1 -> Cross Product1/2

== system detumbling1/Control system/Spin rate damping (MT)/Ideal control law ==
  estW : Inport
  estB_b : Inport  Port=2
  estMd : Inport  Port=3
  Add : Sum  Inputs=+-
  Cross Product : vrlib/Utilities/Cross Product
  Cross Product1 : vrlib/Utilities/Cross Product
  Gain : Gain  Gain=-detumblingkb
  targetMc : Outport
  wires:
  estMd/1 -> Add/2
  Add/1 -> targetMc/1
  Cross Product/1 -> Gain/1
  estB_b/1 -> Cross Product/1, Cross Product1/2
  estW/1 -> Cross Product/2
  Gain/1 -> Cross Product1/1
  Cross Product1/1 -> Add/1

== system detumbling1/Control system/Spin rate damping (MT)/Magnetorquer ==
  targetMc : Inport
  b_b : Inport  Port=2
  estB_b : Inport  Port=3
  Cross Product : vrlib/Utilities/Cross Product
  Cross Product1 : vrlib/Utilities/Cross Product
  Cross Product2 : vrlib/Utilities/Cross Product
  Divide : Product  Inputs=/*
  Dot Product : DotProduct  OutDataTypeStr=Inherit: Inherit via internal rule
  Saturation : Saturate  UpperLimit=maxdipole  LowerLimit=-maxdipole
  Scope : Scope
  Mc_MT : Outport
  estMc_MT : Outport  Port=2
  wires:
  targetMc/1 -> Cross Product/2
  Cross Product/1 -> Divide/2
  Divide/1 -> Saturation/1
  Cross Product1/1 -> Mc_MT/1
  estB_b/1 -> Cross Product2/2, Dot Product/1, Dot Product/2, Cross Product/1
  b_b/1 -> Cross Product1/2
  Saturation/1 -> Scope/1, Cross Product2/1, Cross Product1/1
  Cross Product2/1 -> estMc_MT/1
  Dot Product/1 -> Divide/1

== system detumbling1/External Torques/M_GG/GG Torque1 ==
  c1 : Inport
  c2 : Inport  Port=2
  c3 : Inport  Port=3
  R : Inport  Port=4
  Constant : Constant  Value=3
  Divide : Product  Inputs=*/
  Divide1 : Product  Inputs=*/
  Divide2 : Product  Inputs=*/
  Gain4 : Gain  Gain=3*mu
  Gain5 : Gain  Gain=3*mu
  Gain7 : Gain  Gain=3*mu
  Ix-Iz : Gain  Gain=inertia2
  Iy-Ix : Gain  Gain=inertia3
  Iz-Iy : Gain  Gain=inertia1
  Mux : Mux  Inputs=3
  Pow : Math  Operator=pow  RndMeth=Zero
  Product3 : Product
  Product4 : Product
  Product5 : Product
  M_GG : Outport
  wires:
  Pow/1 -> Divide2/2, Divide1/2, Divide/2
  Iz-Iy/1 -> Mux/1
  c3/1 -> Product3/2, Product4/2
  Product3/1 -> Gain4/1
  Divide2/1 -> Iy-Ix/1
  Gain4/1 -> Divide/1
  Gain5/1 -> Divide1/1
  Divide/1 -> Iz-Iy/1
  Constant/1 -> Pow/2
  Divide1/1 -> Ix-Iz/1
  Product5/1 -> Gain7/1
  c1/1 -> Product5/1, Product4/1
  R/1 -> Pow/1
  Iy-Ix/1 -> Mux/3
  Ix-Iz/1 -> Mux/2
  Gain7/1 -> Divide2/1
  Product4/1 -> Gain5/1
  c2/1 -> Product3/1, Product5/2
  Mux/1 -> M_GG/1

== system detumbling1/External Torques/M_GG/c1, c2, c3 ==
  A_BL : Inport
  Constant1 : Constant  Value=[1; 0; 0]
  Demux : Demux  Outputs=3
  Product1 : Product  Multiplication=Matrix(*)
  c1 : Outport
  c2 : Outport  Port=2
  c3 : Outport  Port=3
  wires:
  Demux/2 -> c2/1
  Product1/1 -> Demux/1
  Demux/1 -> c1/1
  Demux/3 -> c3/1
  Constant1/1 -> Product1/2
  A_BL/1 -> Product1/1

== system detumbling1/External Torques/Solar radiation/Areas ==
  MB : Inport
  Demux : Demux
  Mux : Mux  Inputs=3
  Product1 : Product
  Product2 : Product
  Product4 : Product
  Reshape : Reshape  OutputDimensionality=Column vector (2-D)
  Terminator : Terminator
  A_vect : Outport
  wires:
  Product2/1 -> Mux/2  "a*h"
  Product4/1 -> Mux/1  "b*h"
  MB/1 -> Demux/1
  Product1/1 -> Mux/3  "a*b"
  Demux/1 -> Terminator/1
  Demux/2 -> [a]
  Demux/3 -> [b]
  Demux/4 -> [h]
  [b] -> Product4/1
  [h] -> Product4/2
  [h] -> Product2/2
  [b] -> Product1/2
  [a] -> Product2/1
  [a] -> Product1/1
  Mux/1 -> Reshape/1
  Reshape/1 -> A_vect/1

== system detumbling1/External Torques/Solar radiation/Areas_SP ==
  SP : Inport
  Demux : Demux
  Product1 : Product
  Terminator : Terminator
  Terminator1 : Terminator
  A_vect : Outport
  wires:
  [a] -> Product1/1
  [b] -> Product1/2
  Demux/4 -> Terminator1/1
  Demux/3 -> [b]
  Demux/2 -> [a]
  Demux/1 -> Terminator/1
  Product1/1 -> A_vect/1  "a*b"
  SP/1 -> Demux/1

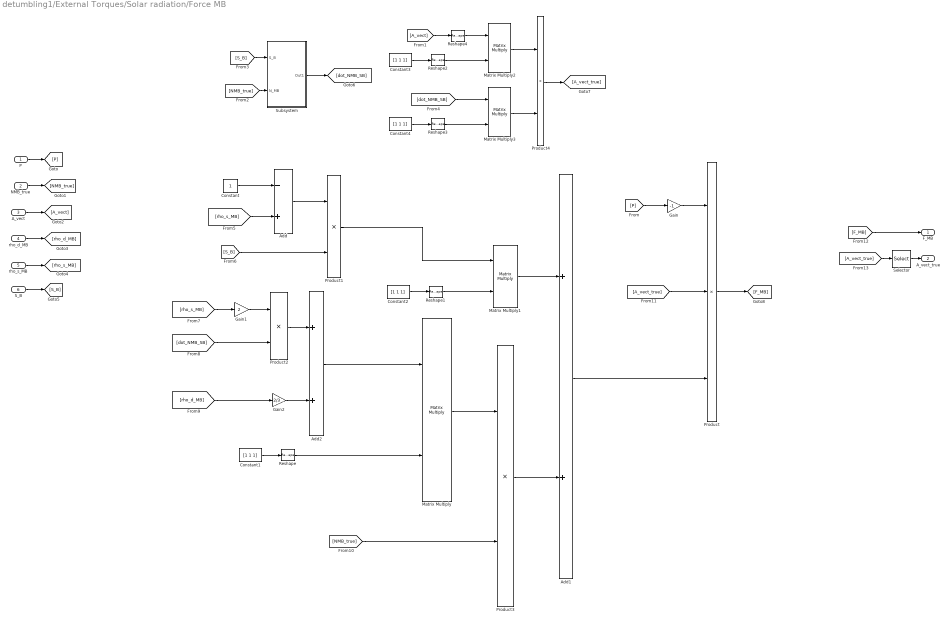
== system detumbling1/External Torques/Solar radiation/Force MB ==
  P : Inport
  NMB_true : Inport  Port=2
  A_vect : Inport  Port=3
  rho_d_MB : Inport  Port=4
  rho_s_MB : Inport  Port=5
  S_B : Inport  Port=6
  Add : Sum  Inputs=-+
  Add1 : Sum
  Add2 : Sum
  Constant : Constant
  Constant{1..4} (4 alike) : Constant  Value=[1 1 1]
  Gain : Gain  Gain=-1
  Gain1 : Gain  Gain=2
  Gain2 : Gain  Gain=2/3
  Matrix Multiply{,1..3} (4 alike) : Product  Multiplication=Matrix(*)
  Product : Product  Inputs=3
  Product{1..4} (4 alike) : Product
  Reshape{,1..3} (4 alike) : Reshape  OutputDimensionality=Row vector (2-D)
  Reshape4 : Reshape  OutputDimensionality=Column vector (2-D)
  Selector : Selector  NumberOfDimensions=2  InputPortWidth=3  IndexOptions=Index vector (dialog),Index vector (dialog)  Indices=[1 2 3],1  OutputSizes=1,1
  Subsystem : Subsystem
  F_MB : Outport
  A_vect_true : Outport  Port=2
  wires:
  P/1 -> [P]
  NMB_true/1 -> [NMB_true]
  A_vect/1 -> [A_vect]
  rho_d_MB/1 -> [rho_d_MB]
  rho_s_MB/1 -> [rho_s_MB]
  S_B/1 -> [S_B]
  [P] -> Gain/1
  Gain/1 -> Product/1
  [NMB_true] -> Subsystem/2(N_MB)
  [S_B] -> Subsystem/1(S_B)
  Subsystem/1(Out1) -> [dot_NMB_SB]
  [rho_s_MB] -> Add/2
  Constant/1 -> Add/1
  Add/1 -> Product1/1
  [S_B] -> Product1/2
  [rho_s_MB] -> Gain1/1
  [dot_NMB_SB] -> Product2/2
  Gain1/1 -> Product2/1
  Product2/1 -> Add2/1
  Gain2/1 -> Add2/2
  [rho_d_MB] -> Gain2/1
  [NMB_true] -> Product3/2
  Product3/1 -> Add1/2
  Add1/1 -> Product/3
  Constant1/1 -> Reshape/1
  Matrix Multiply/1 -> Product3/1
  Add2/1 -> Matrix Multiply/1
  Reshape/1 -> Matrix Multiply/2
  Matrix Multiply1/1 -> Add1/1
  Product1/1 -> Matrix Multiply1/1
  Constant2/1 -> Reshape1/1
  Reshape1/1 -> Matrix Multiply1/2
  Reshape2/1 -> Matrix Multiply2/2
  Constant3/1 -> Reshape2/1
  Reshape3/1 -> Matrix Multiply3/2
  Constant4/1 -> Reshape3/1
  [A_vect] -> Reshape4/1
  Reshape4/1 -> Matrix Multiply2/1
  [dot_NMB_SB] -> Matrix Multiply3/1
  Matrix Multiply2/1 -> Product4/1
  Matrix Multiply3/1 -> Product4/2
  Product4/1 -> [A_vect_true]
  [A_vect_true] -> Product/2
  Product/1 -> [F_MB]
  [F_MB] -> F_MB/1
  [A_vect_true] -> Selector/1
  Selector/1 -> A_vect_true/1

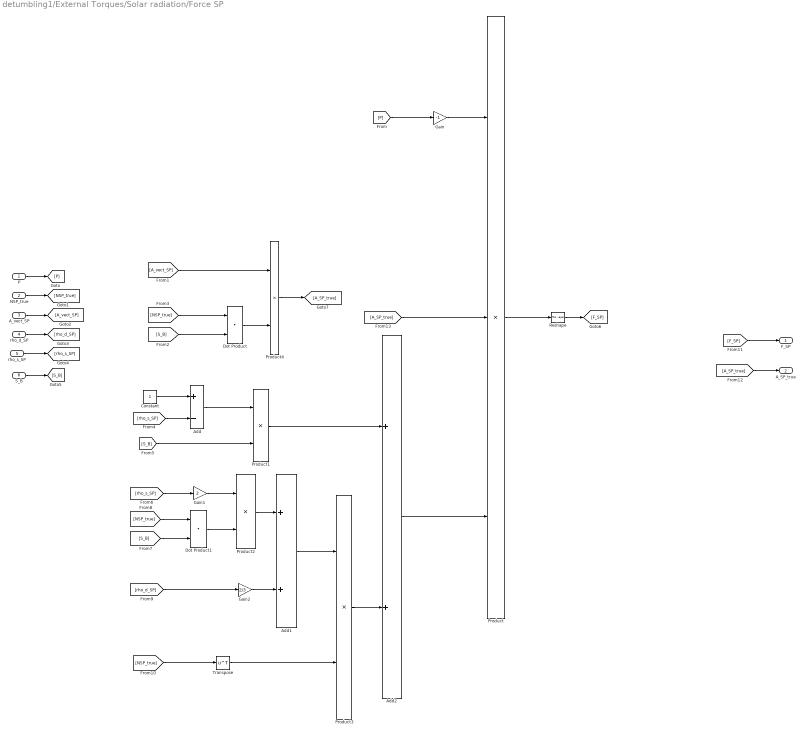
== system detumbling1/External Torques/Solar radiation/Force SP ==
  P : Inport
  NSP_true : Inport  Port=2
  A_vect_SP : Inport  Port=3
  rho_d_SP : Inport  Port=4
  rho_s_SP : Inport  Port=5
  S_B : Inport  Port=6
  Add : Sum  Inputs=+-
  Add1 : Sum
  Add2 : Sum
  Constant : Constant
  Dot Product : DotProduct  OutDataTypeStr=Inherit: Inherit via internal rule
  Dot Product1 : DotProduct  OutDataTypeStr=Inherit: Inherit via internal rule
  Gain : Gain  Gain=-1
  Gain1 : Gain  Gain=2
  Gain2 : Gain  Gain=2/3
  Product : Product  Inputs=3
  Product{1..4} (4 alike) : Product
  Reshape : Reshape  OutputDimensionality=Row vector (2-D)
  Transpose : Math  Operator=transpose
  F_SP : Outport
  A_SP_true : Outport  Port=2
  wires:
  P/1 -> [P]
  NSP_true/1 -> [NSP_true]
  A_vect_SP/1 -> [A_vect_SP]
  rho_d_SP/1 -> [rho_d_SP]
  rho_s_SP/1 -> [rho_s_SP]
  S_B/1 -> [S_B]
  Product/1 -> Reshape/1
  [P] -> Gain/1
  Gain/1 -> Product/1
  [S_B] -> Dot Product/2
  [NSP_true] -> Dot Product/1
  Constant/1 -> Add/1
  [rho_s_SP] -> Add/2
  Add/1 -> Product1/1
  [S_B] -> Product1/2
  [rho_s_SP] -> Gain1/1
  [NSP_true] -> Dot Product1/1
  [S_B] -> Dot Product1/2
  Dot Product1/1 -> Product2/2
  Gain1/1 -> Product2/1
  Product2/1 -> Add1/1
  [rho_d_SP] -> Gain2/1
  Gain2/1 -> Add1/2
  [NSP_true] -> Transpose/1
  Add1/1 -> Product3/1
  Product1/1 -> Add2/1
  Product3/1 -> Add2/2
  Transpose/1 -> Product3/2
  Add2/1 -> Product/3
  Reshape/1 -> [F_SP]
  [F_SP] -> F_SP/1
  Dot Product/1 -> Product4/2
  [A_vect_SP] -> Product4/1
  Product4/1 -> [A_SP_true]
  [A_SP_true] -> A_SP_true/1
  [A_SP_true] -> Product/2

== system detumbling1/External Torques/Solar radiation/Inertia matrix ==
  MB : Inport
  SP : Inport  Port=2
  Demux : Demux
  Demux1 : Demux
  Terminator{,1..5} (6 alike) : Terminator
  r_SP : Subsystem
  r_SP1 : Outport
  r_SP2 : Outport  Port=2
  wires:
  [a_MB] -> r_SP/2(a_MB)
  Demux/1 -> Terminator5/1
  SP/1 -> Demux/1
  Demux1/2 -> [a_MB]
  Demux1/3 -> Terminator/1
  Demux1/1 -> Terminator2/1
  Demux1/4 -> Terminator1/1
  MB/1 -> Demux1/1
  Demux/4 -> Terminator3/1
  Demux/2 -> Terminator4/1
  r_SP/2(r_SP2) -> r_SP2/1
  Demux/3 -> [b_SP]
  [b_SP] -> r_SP/1(b_SP)
  r_SP/1(r_SP1) -> r_SP1/1

== system detumbling1/External Torques/Solar radiation/Pressure ==
  Constant6 : Constant  Value=1358
  Constant7 : Constant  Value=c
  Product8 : Product
  Reciprocal : Product  Inputs=/
  P : Outport
  wires:
  Constant6/1 -> Product8/1
  Reciprocal/1 -> Product8/2
  Product8/1 -> P/1
  Constant7/1 -> Reciprocal/1

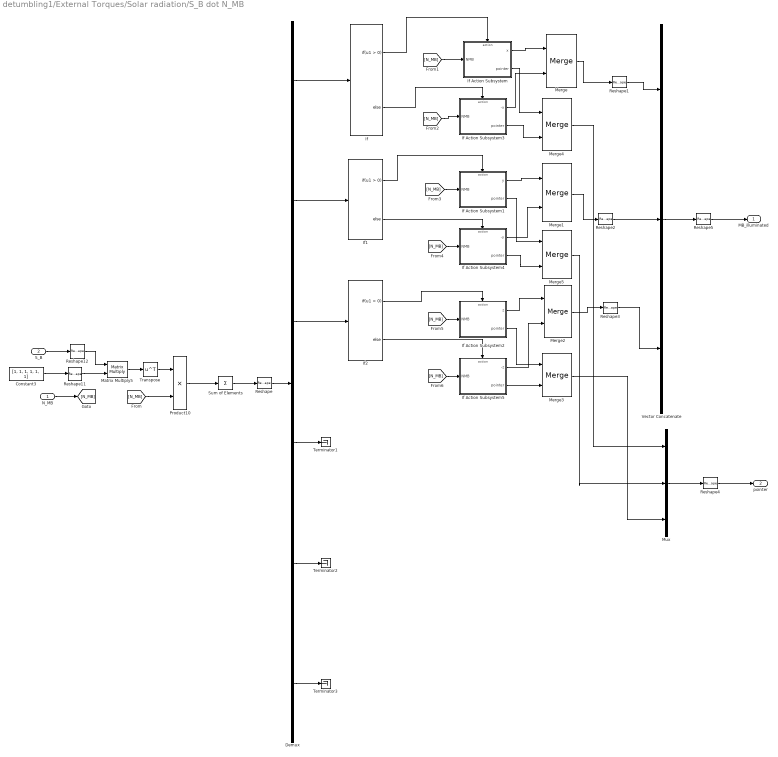
== system detumbling1/External Torques/Solar radiation/S_B dot N_MB ==
  N_MB : Inport
  S_B : Inport  Port=2
  Constant3 : Constant  Value=[1, 1, 1, 1, 1, 1]  VectorParams1D=off
  Demux : Demux  Outputs=6
  If : If
  If Action Subsystem : Subsystem  TreatAsAtomicUnit=on
  If Action Subsystem1 : Subsystem  TreatAsAtomicUnit=on
  If Action Subsystem2 : Subsystem  TreatAsAtomicUnit=on
  If Action Subsystem3 : Subsystem  TreatAsAtomicUnit=on
  If Action Subsystem4 : Subsystem  TreatAsAtomicUnit=on
  If Action Subsystem5 : Subsystem  TreatAsAtomicUnit=on
  If1 : If
  If2 : If
  Matrix Multiply5 : Product  Multiplication=Matrix(*)
  Merge{,1..5} (6 alike) : Merge
  Mux : Mux  Inputs=3
  Product10 : Product
  Reshape{,1..4,12} (6 alike) : Reshape  OutputDimensionality=Column vector (2-D)
  Reshape11 : Reshape  OutputDimensionality=Row vector (2-D)
  Reshape5 : Reshape  OutputDimensionality=Customize  OutputDimensions=[3,3]
  Sum of Elements : Sum  Inputs=+  CollapseMode=Specified dimension  CollapseDim=2
  Terminator1 : Terminator
  Terminator2 : Terminator
  Terminator3 : Terminator
  Transpose : Math  Operator=transpose
  Vector Concatenate : Concatenate  NumInputs=3
  MB_illuminated : Outport
  pointer : Outport  Port=2
  wires:
  Reshape12/1 -> Matrix Multiply5/1
  Matrix Multiply5/1 -> Transpose/1
  Product10/1 -> Sum of Elements/1
  Reshape11/1 -> Matrix Multiply5/2
  Constant3/1 -> Reshape11/1
  S_B/1 -> Reshape12/1
  Sum of Elements/1 -> Reshape/1
  Reshape/1 -> Demux/1
  Demux/1 -> If/1
  If/1 -> If Action Subsystem/Action
  If/2 -> If Action Subsystem3/Action
  N_MB/1 -> [N_MB]
  [N_MB] -> Product10/2
  [N_MB] -> If Action Subsystem/1(NMB)
  Demux/4 -> Terminator1/1
  Demux/5 -> Terminator2/1
  Demux/6 -> Terminator3/1
  Demux/2 -> If1/1
  If1/1 -> If Action Subsystem1/Action
  [N_MB] -> If Action Subsystem3/1(NMB)
  [N_MB] -> If Action Subsystem1/1(NMB)
  If1/2 -> If Action Subsystem4/Action
  [N_MB] -> If Action Subsystem4/1(NMB)
  If Action Subsystem3/1(-x) -> Merge/2
  If Action Subsystem/1(x) -> Merge/1
  If Action Subsystem1/1(y) -> Merge1/1
  If Action Subsystem2/1(z) -> Merge2/1
  If Action Subsystem5/1(-z) -> Merge2/2
  Demux/3 -> If2/1
  If2/1 -> If Action Subsystem2/Action
  If2/2 -> If Action Subsystem5/Action
  [N_MB] -> If Action Subsystem2/1(NMB)
  [N_MB] -> If Action Subsystem5/1(NMB)
  Merge/1 -> Reshape1/1
  Merge1/1 -> Reshape2/1
  Merge2/1 -> Reshape3/1
  Reshape1/1 -> Vector Concatenate/1
  Reshape2/1 -> Vector Concatenate/2
  Reshape3/1 -> Vector Concatenate/3
  Vector Concatenate/1 -> Reshape5/1
  If Action Subsystem4/1(-y) -> Merge1/2
  If Action Subsystem/2(pointer) -> Merge4/1
  If Action Subsystem3/2(pointer) -> Merge4/2
  If Action Subsystem1/2(pointer) -> Merge5/1
  If Action Subsystem4/2(pointer) -> Merge5/2
  If Action Subsystem2/2(pointer) -> Merge3/1
  If Action Subsystem5/2(pointer) -> Merge3/2
  Merge4/1 -> Mux/1
  Merge5/1 -> Mux/2
  Merge3/1 -> Mux/3
  Mux/1 -> Reshape4/1
  Reshape4/1 -> pointer/1
  Reshape5/1 -> MB_illuminated/1
  Transpose/1 -> Product10/1

== system detumbling1/External Torques/Solar radiation/S_B dot N_SP ==
  N_SP : Inport
  S_B : Inport  Port=2
  Constant3 : Constant  Value=[1, 1]
  Demux : Demux  Outputs=2
  If : If
  If Action Subsystem : Subsystem  TreatAsAtomicUnit=on
  If Action Subsystem1 : Subsystem  TreatAsAtomicUnit=on
  If1 : If
  Matrix Multiply5 : Product  Multiplication=Matrix(*)
  Merge : Merge
  Merge1 : Merge
  Product10 : Product
  Reshape11 : Reshape  OutputDimensionality=Row vector (2-D)
  Reshape12 : Reshape  OutputDimensionality=Column vector (2-D)
  Sum of Elements : Sum  Inputs=+  CollapseMode=Specified dimension  CollapseDim=2
  Terminator : Terminator
  Terminator1 : Terminator
  Transpose : Math  Operator=transpose
  SP_illuminated : Outport
  pointer : Outport  Port=2
  wires:
  [N_SP] -> Product10/2
  N_SP/1 -> [N_SP]
  Sum of Elements/1 -> Demux/1
  S_B/1 -> Reshape12/1
  Constant3/1 -> Reshape11/1
  Reshape11/1 -> Matrix Multiply5/2
  Product10/1 -> Sum of Elements/1
  Matrix Multiply5/1 -> Transpose/1
  Reshape12/1 -> Matrix Multiply5/1
  Transpose/1 -> Product10/1
  Demux/1 -> If/1
  If/1 -> If Action Subsystem/Action
  Demux/2 -> If1/1
  [N_SP] -> If Action Subsystem/1(N_SP)
  [N_SP] -> If Action Subsystem1/1(N_SP)
  If1/1 -> If Action Subsystem1/Action
  If1/2 -> Terminator/1
  If/2 -> Terminator1/1
  If Action Subsystem/1(true_NSP) -> Merge/1
  If Action Subsystem1/1(true_NSP) -> Merge/2
  If Action Subsystem/2(pointer) -> Merge1/1
  If Action Subsystem1/2(pointer) -> Merge1/2
  Merge/1 -> SP_illuminated/1
  Merge1/1 -> pointer/1

== system detumbling1/External Torques/Solar radiation/Sun position ==
  A_B_N : Inport
  Clock : Clock
  Constant : Constant  Value=2*pi
  Constant1 : Constant  Value=365*24*60*60
  Constant2 : Constant  Value=23.45
  Degrees to Radians : simulink_extras/Transformations/Degrees to Radians
  MatrixMultiply : Product  Multiplication=Matrix(*)
  Mux : Mux  Inputs=3
  Product{,1..3} (4 alike) : Product
  Reciprocal : Product  Inputs=1
  Reshape : Reshape  OutputDimensionality=Column vector (2-D)
  Sin : Trigonometry  Operator=cos
  Sin1 : Trigonometry
  Sin2 : Trigonometry  Operator=cos
  Sin3 : Trigonometry
  S_B : Outport
  S_N : Outport  Port=2
  wires:
  Product3/1 -> Mux/3
  Degrees to Radians/1 -> Sin3/1, Sin2/1
  Constant1/1 -> Reciprocal/1
  Sin2/1 -> Product2/2
  Product/1 -> Product1/1  "n"
  Constant2/1 -> Degrees to Radians/1
  Product1/1 -> Sin/1, Sin1/1  "n*t"
  Product2/1 -> Mux/2
  Sin3/1 -> Product3/2
  Clock/1 -> Product1/2
  Sin1/1 -> Product3/1, Product2/1
  Constant/1 -> Product/1
  Sin/1 -> Mux/1
  Reciprocal/1 -> Product/2
  Mux/1 -> Reshape/1
  A_B_N/1 -> MatrixMultiply/1
  MatrixMultiply/1 -> S_B/1
  Reshape/1 -> S_N/1, MatrixMultiply/2

== system detumbling1/External Torques/Solar radiation/Torque arm MB ==
  note: creo il vettore somma che ha per colonna i raggi vettori che collegano il CM del MB con i centri illuminati delle facce nel caso che il sole sia nelle 4 posizioni.
  MB : Inport
  A_vect : Inport  Port=2
  S_B : Inport  Port=3
  pointer : Inport  Port=4
  Demux : Demux  Outputs=3
  Reshape : Reshape  OutputDimensionality=Customize  OutputDimensions=[3,3]
  Transpose : Math  Operator=transpose
  Vector Concatenate : Concatenate  NumInputs=3
  creazione raggi vettore tra CM MB e centro facce illuminate della faccia che ha come normale l'asse i : Subsystem
  creazione raggi vettore tra CM MB e centro facce illuminate della faccia che ha come normale l'asse j : Subsystem
  creazione raggi vettore tra CM MB e centro facce illuminate della faccia che ha come normale l'asse k : Subsystem
  dist : Outport
  wires:
  pointer/1 -> Demux/1
  [x] -> creazione raggi vettore tra CM MB e centro facce illuminate della faccia che ha come normale l'asse i/4(pointer)
  [A_vect] -> creazione raggi vettore tra CM MB e centro facce illuminate della faccia che ha come normale l'asse i/3(A_vect)
  [MB] -> creazione raggi vettore tra CM MB e centro facce illuminate della faccia che ha come normale l'asse k/2(MB)
  [y] -> creazione raggi vettore tra CM MB e centro facce illuminate della faccia che ha come normale l'asse j/4(pointer)
  S_B/1 -> [S_B]
  [A_vect] -> creazione raggi vettore tra CM MB e centro facce illuminate della faccia che ha come normale l'asse k/3(A_vect)
  [MB] -> creazione raggi vettore tra CM MB e centro facce illuminate della faccia che ha come normale l'asse j/2(MB)
  A_vect/1 -> [A_vect]
  MB/1 -> [MB]
  [MB] -> creazione raggi vettore tra CM MB e centro facce illuminate della faccia che ha come normale l'asse i/2(MB)
  Reshape/1 -> Transpose/1
  Transpose/1 -> dist/1
  [S_B] -> creazione raggi vettore tra CM MB e centro facce illuminate della faccia che ha come normale l'asse k/1(S_B)
  Demux/1 -> [x]
  Demux/3 -> [z]
  [S_B] -> creazione raggi vettore tra CM MB e centro facce illuminate della faccia che ha come normale l'asse j/1(S_B)
  [z] -> creazione raggi vettore tra CM MB e centro facce illuminate della faccia che ha come normale l'asse k/4(pointer)
  Vector Concatenate/1 -> Reshape/1  "vectors x, y, z"
  [A_vect] -> creazione raggi vettore tra CM MB e centro facce illuminate della faccia che ha come normale l'asse j/3(A_vect)
  [S_B] -> creazione raggi vettore tra CM MB e centro facce illuminate della faccia che ha come normale l'asse i/1(S_B)
  Demux/2 -> [y]
  creazione raggi vettore tra CM MB e centro facce illuminate della faccia che ha come normale l'asse k/1(Out1) -> Vector Concatenate/3
  creazione raggi vettore tra CM MB e centro facce illuminate della faccia che ha come normale l'asse j/1(Out1) -> Vector Concatenate/2
  creazione raggi vettore tra CM MB e centro facce illuminate della faccia che ha come normale l'asse i/1(Out1) -> Vector Concatenate/1
